simulink model "lock_srw_vA_mac"  (R2019a)
settings: Solver=VariableStepAuto  StartTime=0.0  StopTime=inf  RelTol=1e-3
undefined symbols (not defined in the file): f
libraries: dspnetwork x9, instrumentlib x9, simulink x2
(part 1 of 2)
settings Model: EnablePacing=on  PacingRate=200  Creator=SueAnne  LastModifiedBy=sheltonwright
settings DataIOCC: ReturnWorkspaceOutputs=off
settings DebuggingCC: PregeneratedLibrarySubsystemCodeDiagnostic=none  ArithmeticOperatorsInVariantConditions=warning
settings SFSimCC: SimUseLocalCustomCode=off
settings RTWCC: RTWUseLocalCustomCode=off

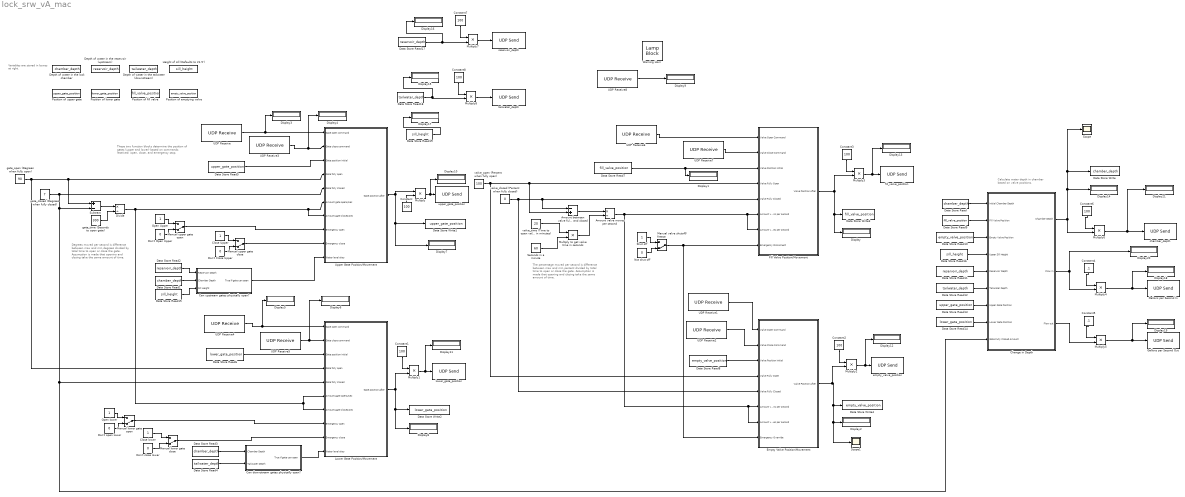
== system lock_srw_vA_mac ==
  note: These two function blocks determine the position of gates (upper and lower) based on commands received: open, close, and emergency stop.
  note: Variables are stored in boxes at right.
  note: Calculate water depth in chamber based on valve positions.
  note: Degrees moved per second is difference between max and min degrees divided by total time to open or close the gate. Assumption is made that opening and closing take the same amount of time.
  note: The percentage moved per second is difference between max and min percent divided by total time to open or close the gate. Assumption is made that opening and closing take the same amount of time.
  Amount between valve fully open and closed : Sum  Inputs=-+  OutDataTypeStr=uint8
  Amount valve moves per second : Product  Inputs=*/  OutDataTypeStr=double
  Can downstream gates physically open? : Subsystem
  Can upstream gates physically open? : Subsystem
  Change in Depth : Subsystem
  Close Upper : Constant
  Close lower : Constant
  Constant{,1..3,6..8} (7 alike) : Constant  Value=100
  Constant4 : Constant  Value=.1
  Constant5 : Constant  Value=.1
  Data Store Read : DataStoreRead  DataStoreName=chamber_depth
  Data Store Read1 : DataStoreRead  Priority=0  DataStoreName=chamber_depth
  Data Store Read10 : DataStoreRead  DataStoreName=empty_valve_position
  Data Store Read11 : DataStoreRead  DataStoreName=reservoir_depth
  Data Store Read12 : DataStoreRead  DataStoreName=tailwater_depth
  Data Store Read13 : DataStoreRead  DataStoreName=upper_gate_position
  Data Store Read14 : DataStoreRead  DataStoreName=lower_gate_position
  Data Store Read15 : DataStoreRead  Priority=0  DataStoreName=sill_height
  Data Store Read16 : DataStoreRead  Priority=0  DataStoreName=sill_height
  Data Store Read17 : DataStoreRead  Priority=0  DataStoreName=reservoir_depth
  Data Store Read18 : DataStoreRead  Priority=0  DataStoreName=tailwater_depth
  Data Store Read19 : DataStoreRead  Priority=0  DataStoreName=sill_height
  Data Store Read2 : DataStoreRead  Priority=0  DataStoreName=reservoir_depth
  Data Store Read3 : DataStoreRead  DataStoreName=chamber_depth
  Data Store Read4 : DataStoreRead  DataStoreName=tailwater_depth
  Data Store Read5 : DataStoreRead  Priority=0  DataStoreName=upper_gate_position
  Data Store Read6 : DataStoreRead  Priority=0  DataStoreName=lower_gate_position
  Data Store Read7 : DataStoreRead  Priority=0  DataStoreName=fill_valve_position
  Data Store Read8 : DataStoreRead  Priority=0  DataStoreName=empty_valve_position
  Data Store Read9 : DataStoreRead  DataStoreName=fill_valve_position
  Data Store Write : DataStoreWrite  DataStoreName=chamber_depth
  Data Store Write1 : DataStoreWrite  Priority=9  DataStoreName=upper_gate_position
  Data Store Write2 : DataStoreWrite  Priority=9  DataStoreName=lower_gate_position
  Data Store Write3 : DataStoreWrite  Priority=9  DataStoreName=fill_valve_position
  Data Store Write4 : DataStoreWrite  Priority=9  DataStoreName=empty_valve_position
  Depth of water in the lock chamber : DataStoreMemory  DataStoreName=chamber_depth  ReadBeforeWriteMsg=warning  WriteAfterWriteMsg=warning  WriteAfterReadMsg=warning  InitialValue=49.5  ShowAdditionalParam=off
  Depth of water in the reservoir (upstream) : DataStoreMemory  DataStoreName=reservoir_depth  ReadBeforeWriteMsg=warning  WriteAfterWriteMsg=warning  WriteAfterReadMsg=warning  InitialValue=28  ShowAdditionalParam=off
  Depth of water in the tailwater (downstream) : DataStoreMemory  DataStoreName=tailwater_depth  ReadBeforeWriteMsg=warning  WriteAfterWriteMsg=warning  WriteAfterReadMsg=warning  InitialValue=27  ShowAdditionalParam=off
  Display{,1..21} (22 alike) : Display
  Divide : Product  Inputs=*/  OutDataTypeStr=double
  Don't Close Upper : Constant  Value=0
  Don't Open Upper : Constant  Value=0
  Don't close lower : Constant  Value=0
  Don't open lower : Constant  Value=0
  Empty Valve Position/Movement : Subsystem
  Fill Valve Position/Movement : Subsystem
  Gallons per Second In : dspnetwork/UDP Send  remoteURL='192.168.56.2'  remotePort=23000  localURL='0.0.0.0'  localPortSource=Automatically determine  localPort=-1  sampletime=-1  blockPlatform=[]  separateLengthPort=0
      settings: SourceProductName=DSP System Toolbox  SourceProductBaseCode=DS
  Gallons per Second Out : dspnetwork/UDP Send  remoteURL='192.168.56.2'  remotePort=23001  localURL='0.0.0.0'  localPortSource=Automatically determine  localPort=-1  sampletime=-1  blockPlatform=[]  separateLengthPort=0
      settings: SourceProductName=DSP System Toolbox  SourceProductBaseCode=DS
  Height of sill (Defaults to 21.5') : DataStoreMemory  DataStoreName=sill_height  ReadBeforeWriteMsg=warning  WriteAfterWriteMsg=warning  WriteAfterReadMsg=warning  InitialValue=21.5  ShowAdditionalParam=off
  Lower Gate Position/Movement : Subsystem
  Manual lower gate close : ManualSwitch  CurrentSetting=0
  Manual lower gate open : ManualSwitch  CurrentSetting=0
  Manual upper gate close : ManualSwitch  CurrentSetting=0
  Manual upper gate open : ManualSwitch  CurrentSetting=0
  Manual valve shutoff/ freeze : ManualSwitch  CurrentSetting=0
  Multiply{,1..8} (9 alike) : Product
  Multiply to get valve time in seconds : Product  OutDataTypeStr=uint16
  Not shut off : Constant  Value=0  OutDataTypeStr=boolean
  Open Upper : Constant
  Open lower : Constant
  Position of emptying valve : DataStoreMemory  DataStoreName=empty_valve_position  ReadBeforeWriteMsg=warning  WriteAfterWriteMsg=warning  WriteAfterReadMsg=warning  ShowAdditionalParam=off
  Position of fill valve : DataStoreMemory  DataStoreName=fill_valve_position  ReadBeforeWriteMsg=warning  WriteAfterWriteMsg=warning  WriteAfterReadMsg=warning  ShowAdditionalParam=off  OutMin=0  OutMax=100  OutDataTypeStr=double
  Position of lower gate : DataStoreMemory  DataStoreName=lower_gate_position  ReadBeforeWriteMsg=warning  WriteAfterWriteMsg=warning  WriteAfterReadMsg=warning  InitialValue=7  ShowAdditionalParam=off
  Position of upper gate : DataStoreMemory  DataStoreName=upper_gate_position  ReadBeforeWriteMsg=warning  WriteAfterWriteMsg=warning  WriteAfterReadMsg=warning  InitialValue=7  ShowAdditionalParam=off
  Scope : Scope
  Scope1 : Scope
  Seconds in a minute : Constant  Value=60  OutDataTypeStr=uint8
  Shut off : Constant  OutDataTypeStr=boolean
  Subtract : Sum  Inputs=+-
  UDP Receive : instrumentlib/UDP Receive  Host=localhost  Port=9090  LocalPort=22000  EnablePortSharing=off  GetLatestData=on  DataSize=[1 1]  DataType=uint16  ASCIIFormatting=%f,  Terminator=LF  ByteOrder=LittleEndian  EnableBlockingMode=on  Timeout=10  SampleTime=1  LocalAddress=192.168.56.1
      settings: SourceProductName=Instrument Control Toolbox
  UDP Receive1 : instrumentlib/UDP Receive  Host=localhost  Port=9090  LocalPort=22006  EnablePortSharing=off  GetLatestData=on  DataSize=[1 1]  DataType=uint16  ASCIIFormatting=%f,  Terminator=LF  ByteOrder=LittleEndian  EnableBlockingMode=on  Timeout=10  SampleTime=1  LocalAddress=192.168.56.1
      settings: SourceProductName=Instrument Control Toolbox
  UDP Receive2 : instrumentlib/UDP Receive  Host=localhost  Port=9090  LocalPort=22007  EnablePortSharing=off  GetLatestData=on  DataSize=[1 1]  DataType=uint16  ASCIIFormatting=%f,  Terminator=LF  ByteOrder=LittleEndian  EnableBlockingMode=on  Timeout=10  SampleTime=1  LocalAddress=192.168.56.1
      settings: SourceProductName=Instrument Control Toolbox
  UDP Receive3 : instrumentlib/UDP Receive  Host=localhost  Port=9090  LocalPort=22001  EnablePortSharing=off  GetLatestData=on  DataSize=[1 1]  DataType=uint16  ASCIIFormatting=%f,  Terminator=LF  ByteOrder=LittleEndian  EnableBlockingMode=on  Timeout=10  SampleTime=1  LocalAddress=192.168.56.1
      settings: SourceProductName=Instrument Control Toolbox
  UDP Receive4 : instrumentlib/UDP Receive  Host=localhost  Port=9090  LocalPort=22002  EnablePortSharing=off  GetLatestData=on  DataSize=[1 1]  DataType=uint16  ASCIIFormatting=%f,  Terminator=LF  ByteOrder=LittleEndian  EnableBlockingMode=on  Timeout=10  SampleTime=1  LocalAddress=192.168.56.1
      settings: SourceProductName=Instrument Control Toolbox
  UDP Receive5 : instrumentlib/UDP Receive  Host=localhost  Port=9090  LocalPort=22003  EnablePortSharing=off  GetLatestData=on  DataSize=[1 1]  DataType=uint16  ASCIIFormatting=%f,  Terminator=LF  ByteOrder=LittleEndian  EnableBlockingMode=on  Timeout=10  SampleTime=1  LocalAddress=192.168.56.1
      settings: SourceProductName=Instrument Control Toolbox
  UDP Receive6 : instrumentlib/UDP Receive  Host=localhost  Port=9090  LocalPort=22004  EnablePortSharing=off  GetLatestData=on  DataSize=[1 1]  DataType=uint16  ASCIIFormatting=%f,  Terminator=LF  ByteOrder=LittleEndian  EnableBlockingMode=on  Timeout=10  SampleTime=1  LocalAddress=192.168.56.1
      settings: SourceProductName=Instrument Control Toolbox
  UDP Receive7 : instrumentlib/UDP Receive  Host=localhost  Port=9090  LocalPort=22005  EnablePortSharing=off  GetLatestData=on  DataSize=[1 1]  DataType=uint16  ASCIIFormatting=%f,  Terminator=LF  ByteOrder=LittleEndian  EnableBlockingMode=on  Timeout=10  SampleTime=1  LocalAddress=192.168.56.1
      settings: SourceProductName=Instrument Control Toolbox
  UDP Receive8 : instrumentlib/UDP Receive  Host=localhost  Port=9090  LocalPort=22010  EnablePortSharing=off  GetLatestData=on  DataSize=[1 1]  DataType=uint16  ASCIIFormatting=%f,  Terminator=LF  ByteOrder=LittleEndian  EnableBlockingMode=on  Timeout=10  SampleTime=1  LocalAddress=192.168.56.1
      settings: SourceProductName=Instrument Control Toolbox
  Upper Gate Position/Movement : Subsystem
  Warning Horn : LampBlock
  chamber_depth : dspnetwork/UDP Send  remoteURL='192.168.56.2'  remotePort=23006  localURL='0.0.0.0'  localPortSource=Automatically determine  localPort=-1  sampletime=-1  blockPlatform=[]  separateLengthPort=0
      settings: SourceProductName=DSP System Toolbox  SourceProductBaseCode=DS
  empty_valve_position : dspnetwork/UDP Send  remoteURL='192.168.56.2'  remotePort=23005  localURL='0.0.0.0'  localPortSource=Automatically determine  localPort=-1  sampletime=-1  blockPlatform=[]  separateLengthPort=0
      settings: SourceProductName=DSP System Toolbox  SourceProductBaseCode=DS
  fill_valve_position : dspnetwork/UDP Send  remoteURL='192.168.56.2'  remotePort=23004  localURL='0.0.0.0'  localPortSource=Automatically determine  localPort=-1  sampletime=-1  blockPlatform=[]  separateLengthPort=0
      settings: SourceProductName=DSP System Toolbox  SourceProductBaseCode=DS
  gate_closed (Degrees when fully closed) : Constant  Value=7
  gate_open (Degrees when fully open) : Constant  Value=90
  gate_time (Seconds to open gate) : Constant  Value=300
  lower_gate_position : dspnetwork/UDP Send  remoteURL='192.168.56.2'  remotePort=23003  localURL='0.0.0.0'  localPortSource=Automatically determine  localPort=-1  sampletime=-1  blockPlatform=[]  separateLengthPort=0
      settings: SourceProductName=DSP System Toolbox  SourceProductBaseCode=DS
  reservoir_depth : dspnetwork/UDP Send  remoteURL='192.168.56.2'  remotePort=23007  localURL='0.0.0.0'  localPortSource=Automatically determine  localPort=-1  sampletime=-1  blockPlatform=[]  separateLengthPort=0
      settings: SourceProductName=DSP System Toolbox  SourceProductBaseCode=DS
  tailwater_depth : dspnetwork/UDP Send  remoteURL='192.168.56.2'  remotePort=23008  localURL='0.0.0.0'  localPortSource=Automatically determine  localPort=-1  sampletime=-1  blockPlatform=[]  separateLengthPort=0
      settings: SourceProductName=DSP System Toolbox  SourceProductBaseCode=DS
  upper_gate_position : dspnetwork/UDP Send  remoteURL='192.168.56.2'  remotePort=23002  localURL='0.0.0.0'  localPortSource=Automatically determine  localPort=-1  sampletime=-1  blockPlatform=[]  separateLengthPort=0
      settings: SourceProductName=DSP System Toolbox  SourceProductBaseCode=DS
  valve_closed (Percent when fully closed) : Constant  Value=0  OutDataTypeStr=uint8
  valve_open (Percent when fully open) : Constant  Value=100  OutDataTypeStr=uint8
  "valve_time (Time to open valve, in minutes)" : Constant  Value=20  OutDataTypeStr=uint8
  wires:
  UDP Receive/1 -> Display3/1, Upper Gate Position/Movement/1(Gate open command)
  UDP Receive3/1 -> Display4/1, Upper Gate Position/Movement/2(Gate close command)
  gate_open (Degrees when fully open)/1 -> Lower Gate Position/Movement/4(Gate fully open), Subtract/1, Upper Gate Position/Movement/4(Gate fully open)
  gate_closed (Degrees when fully closed)/1 -> Change in Depth/9(Gate Fully Closed Amount), Lower Gate Position/Movement/5(Gate fully closed), Subtract/2, Upper Gate Position/Movement/5(Gate fully closed)
  Manual upper gate open/1 -> Upper Gate Position/Movement/8(Emergency open)
  Data Store Read/1 -> Change in Depth/1(Initial Chamber Depth)
  Change in Depth/1(Chamber Depth) -> Multiply6/2, Scope/1, Data Store Write/1, Display14/1
  Lower Gate Position/Movement/1(Gate position after) -> Multiply1/2, Data Store Write2/1, Display8/1
  UDP Receive4/1 -> Lower Gate Position/Movement/1(Gate open command), Display5/1
  Can upstream gates physically open?/1(True if gate can open) -> Upper Gate Position/Movement/10(Water level okay)
  Data Store Read4/1 -> Can downstream gates physically open?/2(Tailwater Depth)
  Data Store Read3/1 -> Can downstream gates physically open?/1(Chamber Depth)
  Data Store Read1/1 -> Can upstream gates physically open?/2(Chamber Depth)
  Data Store Read5/1 -> Upper Gate Position/Movement/3(Gate position initial)
  Data Store Read6/1 -> Lower Gate Position/Movement/3(Gate position initial)
  gate_time (Seconds to open gate)/1 -> Divide/2
  Subtract/1 -> Divide/1
  Divide/1 -> Lower Gate Position/Movement/7(Amount gate closes/sec), Lower Gate Position/Movement/6(Amount gate opens/sec), Upper Gate Position/Movement/7(Amount gate closes/sec), Upper Gate Position/Movement/6(Amount gate opens/sec)
  Data Store Read7/1 -> Display1/1, Fill Valve Position/Movement/3(Valve Position Initial)
  valve_open (Percent when fully open)/1 -> Amount between valve fully open and closed/2, Fill Valve Position/Movement/4(Valve Fully Open), Empty Valve Position/Movement/4(Valve Fully Open)
  valve_closed (Percent when fully closed)/1 -> Fill Valve Position/Movement/5(Valve Fully Closed), Amount between valve fully open and closed/1, Empty Valve Position/Movement/5(Valve Fully Closed)
  Manual valve shutoff/ freeze/1 -> Fill Valve Position/Movement/8(Emergency Disconnect), Empty Valve Position/Movement/8(Emergency Override)
  "valve_time (Time to open valve, in minutes)"/1 -> Multiply to get valve time in seconds/1
  Seconds in a minute/1 -> Multiply to get valve time in seconds/2
  Amount between valve fully open and closed/1 -> Amount valve moves per second/1
  Multiply to get valve time in seconds/1 -> Amount valve moves per second/2
  Amount valve moves per second/1 -> Fill Valve Position/Movement/7(Amount valve closes per second), Fill Valve Position/Movement/6(Amount valve opens per second), Empty Valve Position/Movement/7(Amount valve closes per second), Empty Valve Position/Movement/6(Amount valve opens per second)
  Data Store Read8/1 -> Empty Valve Position/Movement/3(Valve Position Initial)
  Data Store Read9/1 -> Change in Depth/2(Fill Valve Position)
  Data Store Read10/1 -> Change in Depth/3(Empty Valve Position)
  UDP Receive6/1 -> Fill Valve Position/Movement/1(Valve Open Command)
  UDP Receive7/1 -> Fill Valve Position/Movement/2(Valve Close Command)
  UDP Receive1/1 -> Empty Valve Position/Movement/1(Valve Open Command)
  UDP Receive2/1 -> Empty Valve Position/Movement/2(Valve Close Command)
  UDP Receive5/1 -> Lower Gate Position/Movement/2(Gate close command), Display6/1
  Upper Gate Position/Movement/1(Gate position after) -> Multiply/1, Display7/1, Data Store Write1/1
  Multiply/1 -> Display10/1, upper_gate_position/1
  Constant/1 -> Multiply/2
  Multiply1/1 -> Display11/1, lower_gate_position/1
  Constant1/1 -> Multiply1/1
  Constant2/1 -> Multiply2/1
  Empty Valve Position/Movement/1(Valve Position After) -> Multiply2/2, Scope1/1, Display2/1, Data Store Write4/1
  Multiply2/1 -> Display12/1, empty_valve_position/1
  Fill Valve Position/Movement/1(Valve Position After) -> Multiply3/2, Data Store Write3/1, Display/1
  Multiply3/1 -> Display13/1, fill_valve_position/1
  Constant3/1 -> Multiply3/1
  Data Store Read11/1 -> Change in Depth/5(Reservoir Depth)
  Data Store Read16/1 -> Change in Depth/4(Upper Sill Height)
  Data Store Read12/1 -> Change in Depth/6(Tailwater Depth)
  Data Store Read13/1 -> Change in Depth/7(Upper Gate Position)
  Data Store Read14/1 -> Change in Depth/8(Lower Gate Position)
  Data Store Read2/1 -> Can upstream gates physically open?/1(Reservoir Depth)
  Data Store Read15/1 -> Can upstream gates physically open?/3(Sill Height)
  Don't Open Upper/1 -> Manual upper gate open/2
  Open Upper/1 -> Manual upper gate open/1
  Don't Close Upper/1 -> Manual upper gate close/2
  Manual upper gate close/1 -> Upper Gate Position/Movement/9(Emergency close)
  Close Upper/1 -> Manual upper gate close/1
  Can downstream gates physically open?/1(True if gate can open) -> Lower Gate Position/Movement/10(Water level okay)
  Don't open lower/1 -> Manual lower gate open/2
  Manual lower gate open/1 -> Lower Gate Position/Movement/8(Emergency open)
  Manual lower gate close/1 -> Lower Gate Position/Movement/9(Emergency close)
  Open lower/1 -> Manual lower gate open/1
  Close lower/1 -> Manual lower gate close/1
  Don't close lower/1 -> Manual lower gate close/2
  Shut off/1 -> Manual valve shutoff/ freeze/1
  Not shut off/1 -> Manual valve shutoff/ freeze/2
  Change in Depth/2(Flow in) -> Display20/1, Multiply4/2
  Constant4/1 -> Multiply4/1
  Multiply4/1 -> Display18/1, Gallons per Second In/1
  Constant5/1 -> Multiply5/1
  Multiply5/1 -> Display19/1, Gallons per Second Out/1
  Change in Depth/3(Flow out) -> Multiply5/2
  Data Store Read17/1 -> Display16/1, Multiply7/2
  Data Store Read18/1 -> Display15/1, Multiply8/2
  Data Store Read19/1 -> Display17/1
  UDP Receive8/1 -> Display9/1
  Constant6/1 -> Multiply6/1
  Multiply6/1 -> Display21/1, chamber_depth/1
  Constant7/1 -> Multiply7/1
  Multiply7/1 -> reservoir_depth/1
  Constant8/1 -> Multiply8/1
  Multiply8/1 -> tailwater_depth/1

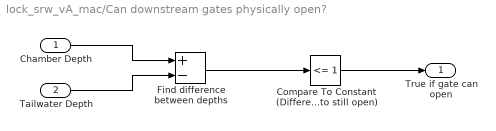
== system lock_srw_vA_mac/Can downstream gates physically open? ==
  Chamber Depth : Inport
  Tailwater Depth : Inport  Port=2
  Compare To Constant (Difference allowed between depths for gate to still open) : simulink/Logic and Bit Operations/Compare To Constant  relop=<=  const=1  OutDataTypeStr=boolean
  Find difference between depths : Sum  Inputs=+-
  True if gate can open : Outport
  wires:
  Chamber Depth/1 -> Find difference between depths/1
  Tailwater Depth/1 -> Find difference between depths/2
  Compare To Constant (Difference allowed between depths for gate to still open)/1 -> True if gate can open/1
  Find difference between depths/1 -> Compare To Constant (Difference allowed between depths for gate to still open)/1

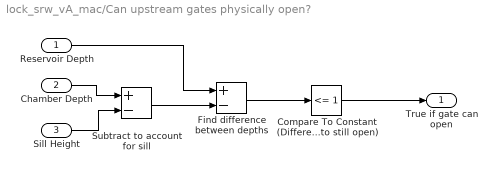
== system lock_srw_vA_mac/Can upstream gates physically open? ==
  Reservoir Depth : Inport
  Chamber Depth : Inport  Port=2
  Sill Height : Inport  Port=3
  Compare To Constant (Difference allowed between depths for gate to still open) : simulink/Logic and Bit Operations/Compare To Constant  relop=<=  const=1  OutDataTypeStr=boolean
  Find difference between depths : Sum  Inputs=+-
  Subtract to account for sill : Sum  Inputs=+-
  True if gate can open : Outport
  wires:
  Compare To Constant (Difference allowed between depths for gate to still open)/1 -> True if gate can open/1
  Find difference between depths/1 -> Compare To Constant (Difference allowed between depths for gate to still open)/1
  Subtract to account for sill/1 -> Find difference between depths/2
  Chamber Depth/1 -> Subtract to account for sill/1
  Sill Height/1 -> Subtract to account for sill/2
  Reservoir Depth/1 -> Find difference between depths/1

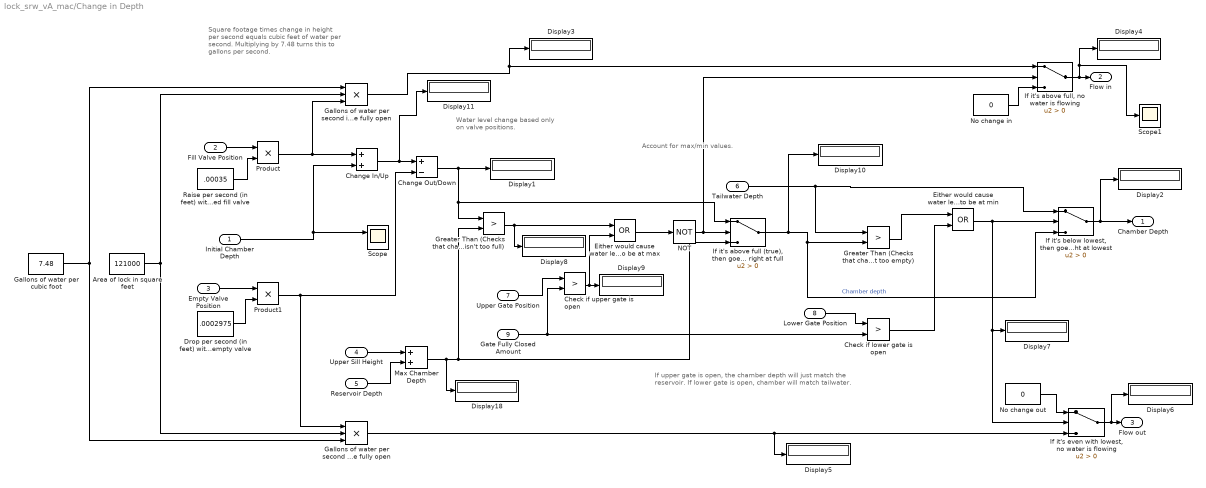
== system lock_srw_vA_mac/Change in Depth ==
  note: If upper gate is open, the chamber depth will just match the reservoir. If lower gate is open, chamber will match tailwater.
  note: Water level change based only on valve positions.
  note: Account for max/min values.
  note: Square footage times change in height per second equals cubic feet of water per second. Multiplying by 7.48 turns this to gallons per second.
  Initial Chamber Depth : Inport
  Fill Valve Position : Inport  Port=2
  Empty Valve Position : Inport  Port=3
  Upper Sill Height : Inport  Port=4
  Reservoir Depth : Inport  Port=5
  Tailwater Depth : Inport  Port=6
  Upper Gate Position : Inport  Port=7
  Lower Gate Position : Inport  Port=8
  Gate Fully Closed Amount : Inport  Port=9
  Area of lock in square feet : Constant  Value=121000  OutDataTypeStr=double
  Change Out/Down : Sum  Inputs=+-
  Change In/Up : Sum
  Check if lower gate is open : RelationalOperator  Operator=>  OutDataTypeStr=boolean  RndMeth=Simplest
  Check if upper gate is open : RelationalOperator  Operator=>  OutDataTypeStr=boolean  RndMeth=Simplest
  Display{1..11,18} (12 alike) : Display
  Drop per second (in feet) with fully opened empty valve : Constant  Value=.0002975  OutDataTypeStr=double
  Either would cause water level to be at max : Logic  Operator=OR  AllPortsSameDT=off  OutDataTypeStr=boolean
  Either would cause water level to be at min : Logic  Operator=OR  AllPortsSameDT=off  OutDataTypeStr=boolean
  Gallons of water per cubic foot : Constant  Value=7.48  OutDataTypeStr=double
  "Gallons of water per second in, when fill valve fully open" : Product  Inputs=3
  "Gallons of water per second out, when empty valve fully open" : Product  Inputs=3
  Greater Than (Checks that chamber isn't too empty) : RelationalOperator  Operator=>  OutDataTypeStr=boolean  RndMeth=Simplest
  Greater Than (Checks that chamber isn't too full) : RelationalOperator  Operator=>  OutDataTypeStr=boolean  RndMeth=Simplest
  "If it's above full (true), then goes back to being right at full" : Switch  Criteria=u2 > Threshold
  "If it's above full, no water is flowing" : Switch  Criteria=u2 > Threshold
  "If it's below lowest, then goes back to being right at lowest" : Switch  Criteria=u2 > Threshold
  "If it's even with lowest, no water is flowing" : Switch  Criteria=u2 > Threshold
  Max Chamber Depth : Sum
  NOT : Logic  Operator=NOT  IconShape=distinctive  AllPortsSameDT=off  OutDataTypeStr=boolean
  No change in : Constant  Value=0  OutDataTypeStr=double
  No change out : Constant  Value=0  OutDataTypeStr=double
  Product : Product
  Product1 : Product
  Raise per second (in feet) with fully opened fill valve : Constant  Value=.00035  OutDataTypeStr=double
  Scope : Scope  NumInputPorts=2
  Scope1 : Scope
  Chamber Depth : Outport
  Flow in : Outport  Port=2
  Flow out : Outport  Port=3
  wires:
  Fill Valve Position/1 -> Product/1
  Product/1 -> "Gallons of water per second in, when fill valve fully open"/3, Change In/Up/1
  Change In/Up/1 -> Display11/1, Change Out/Down/1
  Empty Valve Position/1 -> Product1/1
  Product1/1 -> "Gallons of water per second out, when empty valve fully open"/1, Change Out/Down/2
  Upper Sill Height/1 -> Max Chamber Depth/1
  Reservoir Depth/1 -> Max Chamber Depth/2
  Max Chamber Depth/1 -> Display18/1, Greater Than (Checks that chamber isn't too full)/2, "If it's above full (true), then goes back to being right at full"/3
  Change Out/Down/1 -> "If it's above full (true), then goes back to being right at full"/1, Greater Than (Checks that chamber isn't too full)/1, Display1/1
  "If it's above full (true), then goes back to being right at full"/1 -> Display10/1, Greater Than (Checks that chamber isn't too empty)/2, "If it's below lowest, then goes back to being right at lowest"/3  "Chamber depth"
  Greater Than (Checks that chamber isn't too full)/1 -> Either would cause water level to be at max/1, Display8/1
  Upper Gate Position/1 -> Check if upper gate is open/1
  Gate Fully Closed Amount/1 -> Check if upper gate is open/2, Check if lower gate is open/2
  Greater Than (Checks that chamber isn't too empty)/1 -> Either would cause water level to be at min/1
  Either would cause water level to be at min/1 -> Display7/1, "If it's even with lowest, no water is flowing"/2, "If it's below lowest, then goes back to being right at lowest"/2
  Lower Gate Position/1 -> Check if lower gate is open/1
  "If it's below lowest, then goes back to being right at lowest"/1 -> Display2/1, Chamber Depth/1
  Check if upper gate is open/1 -> Either would cause water level to be at max/2, Display9/1
  Gallons of water per cubic foot/1 -> "Gallons of water per second in, when fill valve fully open"/1, "Gallons of water per second out, when empty valve fully open"/3
  Initial Chamber Depth/1 -> Scope/1, Change In/Up/2
  Drop per second (in feet) with fully opened empty valve/1 -> Product1/2
  Raise per second (in feet) with fully opened fill valve/1 -> Product/2
  Area of lock in square feet/1 -> "Gallons of water per second out, when empty valve fully open"/2, "Gallons of water per second in, when fill valve fully open"/2
  "Gallons of water per second in, when fill valve fully open"/1 -> "If it's above full, no water is flowing"/1, Display3/1
  "If it's above full, no water is flowing"/1 -> Display4/1, Scope1/1, Flow in/1
  No change in/1 -> "If it's above full, no water is flowing"/3
  "If it's even with lowest, no water is flowing"/1 -> Flow out/1, Display6/1
  "Gallons of water per second out, when empty valve fully open"/1 -> Display5/1, "If it's even with lowest, no water is flowing"/3
  Tailwater Depth/1 -> Greater Than (Checks that chamber isn't too empty)/1, "If it's below lowest, then goes back to being right at lowest"/1
  No change out/1 -> "If it's even with lowest, no water is flowing"/1
  Either would cause water level to be at max/1 -> NOT/1
  NOT/1 -> "If it's above full, no water is flowing"/2, "If it's above full (true), then goes back to being right at full"/2
  Check if lower gate is open/1 -> Either would cause water level to be at min/2

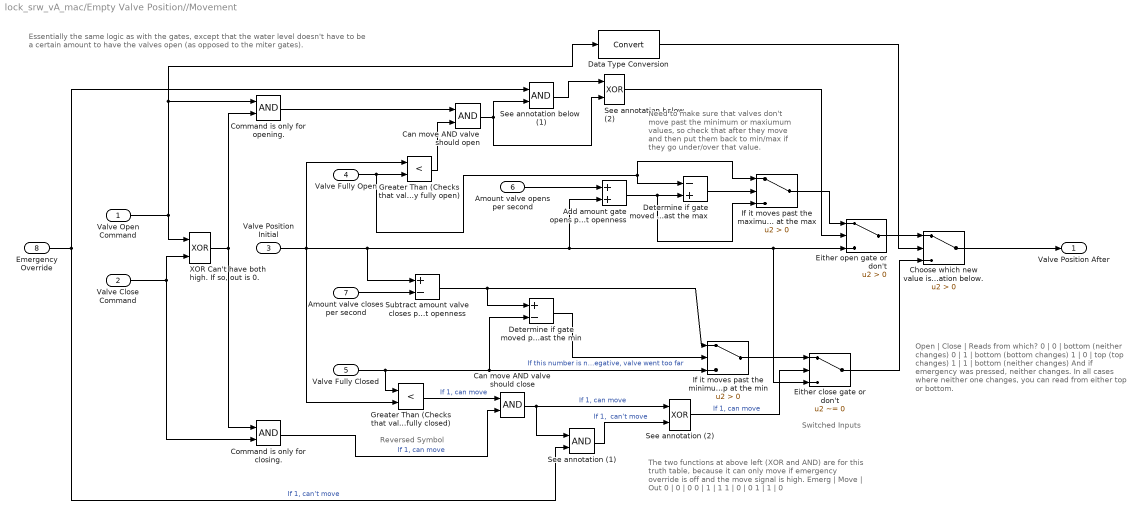
== system lock_srw_vA_mac/Empty Valve Position//Movement ==
  note: Switched Inputs
  note: Reversed Symbol
  note: Essentially the same logic as with the gates, except that the water level doesn't have to be a certain amount to have the valves open (as opposed to the miter gates).
  note: Open	|	Close	|	Reads from which?
      | 0		|	0		|	bottom (neither changes)
      | 0		|	1		|	bottom (bottom changes)
      | 1		|	0		|	top (top changes)
      | 1		|	1		|	bottom (neither changes)
      |
      | And if emergency was pressed, neither changes.  In all cases where neither one changes, you can read from either top or bottom.
  note: The two functions at above left (XOR and AND) are for this truth table, because it can only move if emergency override is off and the move signal is high.
      |
      | Emerg	|	Move	| Out
      | 0		|	0		|	0
      | 0		|	1		|	1
      | 1		|	0		|	0
      | 1		|	1		|	0
  note: Need to make sure that valves don't move past the minimum or maxiumum values, so check that after they move and then put them back to min/max if they go under/over that value.
  Valve Open Command : Inport
  Valve Close Command : Inport  Port=2
  Valve Position Initial : Inport  Port=3
  Valve Fully Open : Inport  Port=4
  Valve Fully Closed : Inport  Port=5
  Amount valve opens per second : Inport  Port=6
  Amount valve closes per second : Inport  Port=7
  Emergency Override : Inport  Port=8
  Add amount gate opens per second to current openness : Sum
  Can move AND valve should close : Logic  AllPortsSameDT=off  OutDataTypeStr=boolean
  Can move AND valve should open : Logic  AllPortsSameDT=off  OutDataTypeStr=boolean
  "Choose which new value is correct, based upon the open command. See annotation below." : Switch  Criteria=u2 > Threshold
  Command is only for closing. : Logic  AllPortsSameDT=off  OutDataTypeStr=boolean
  Command is only for opening. : Logic  AllPortsSameDT=off  OutDataTypeStr=boolean
  Data Type Conversion : DataTypeConversion
  Determine if gate moved past the max : Sum  Inputs=-+
  Determine if gate moved past the min : Sum  Inputs=+-
  Either close gate or don't : Switch  Criteria=u2 ~= 0  RndMeth=Simplest
  Either open gate or don't : Switch  Criteria=u2 > Threshold
  Greater Than (Checks that valve isn't already fully closed) : RelationalOperator  Operator=<  OutDataTypeStr=boolean  RndMeth=Simplest
  Greater Than (Checks that valve isn't already fully open) : RelationalOperator  Operator=<  OutDataTypeStr=boolean  RndMeth=Simplest
  "If it moves past the maximum, it will stop at the max" : Switch  Criteria=u2 > Threshold
  "If it moves past the minimum, it will stop at the min" : Switch  Criteria=u2 > Threshold
  See annotation below  (1) : Logic  AllPortsSameDT=off  OutDataTypeStr=boolean
  See annotation below (2) : Logic  Operator=XOR  IconShape=distinctive  AllPortsSameDT=off  OutDataTypeStr=boolean
  See annotation (1) : Logic  AllPortsSameDT=off  OutDataTypeStr=boolean
  See annotation (2) : Logic  Operator=XOR  IconShape=distinctive  AllPortsSameDT=off  OutDataTypeStr=boolean
  Subtract amount valve closes per second from current openness : Sum  Inputs=+-
  "XOR Can't have both high. If so, out is 0." : Logic  Operator=XOR  IconShape=distinctive  AllPortsSameDT=off  OutDataTypeStr=boolean
  Valve Position After : Outport
  wires:
  Command is only for opening./1 -> Can move AND valve should open/1
  Greater Than (Checks that valve isn't already fully open)/1 -> Can move AND valve should open/2
  Either open gate or don't/1 -> "Choose which new value is correct, based upon the open command. See annotation below."/1
  See annotation (1)/1 -> See annotation (2)/2  "If 1,  can't move"
  Valve Open Command/1 -> Data Type Conversion/1, Command is only for opening./1, "XOR Can't have both high. If so, out is 0."/1
  Valve Fully Open/1 -> Determine if gate moved past the max/1, "If it moves past the maximum, it will stop at the max"/1, Greater Than (Checks that valve isn't already fully open)/2
  "If it moves past the maximum, it will stop at the max"/1 -> Either open gate or don't/1
  Subtract amount valve closes per second from current openness/1 -> "If it moves past the minimum, it will stop at the min"/1, Determine if gate moved past the min/1
  Can move AND valve should open/1 -> See annotation below (2)/2, See annotation below  (1)/2
  Amount valve closes per second/1 -> Subtract amount valve closes per second from current openness/2
  See annotation below  (1)/1 -> See annotation below (2)/1
  Valve Position Initial/1 -> Greater Than (Checks that valve isn't already fully open)/1, Either close gate or don't/3, Either open gate or don't/3, Add amount gate opens per second to current openness/2, Subtract amount valve closes per second from current openness/1, Greater Than (Checks that valve isn't already fully closed)/2
  Either close gate or don't/1 -> "Choose which new value is correct, based upon the open command. See annotation below."/3
  Emergency Override/1 -> See annotation below  (1)/1, See annotation (1)/2  "If 1, can't move"
  See annotation below (2)/1 -> Either open gate or don't/2
  Valve Close Command/1 -> Command is only for closing./2, "XOR Can't have both high. If so, out is 0."/2
  Command is only for closing./1 -> Can move AND valve should close/2  "If 1, can move"
  See annotation (2)/1 -> Either close gate or don't/2  "If 1, can move"
  Can move AND valve should close/1 -> See annotation (2)/1, See annotation (1)/1  "If 1, can move"
  Add amount gate opens per second to current openness/1 -> Determine if gate moved past the max/2, "If it moves past the maximum, it will stop at the max"/3
  Determine if gate moved past the min/1 -> "If it moves past the minimum, it will stop at the min"/2  "If this number is negative, valve went too far"
  Greater Than (Checks that valve isn't already fully closed)/1 -> Can move AND valve should close/1  "If 1, can move"
  Valve Fully Closed/1 -> "If it moves past the minimum, it will stop at the min"/3, Determine if gate moved past the min/2, Greater Than (Checks that valve isn't already fully closed)/1
  Determine if gate moved past the max/1 -> "If it moves past the maximum, it will stop at the max"/2
  "XOR Can't have both high. If so, out is 0."/1 -> Command is only for closing./1, Command is only for opening./2
  Amount valve opens per second/1 -> Add amount gate opens per second to current openness/1
  "Choose which new value is correct, based upon the open command. See annotation below."/1 -> Valve Position After/1
  Data Type Conversion/1 -> "Choose which new value is correct, based upon the open command. See annotation below."/2
  "If it moves past the minimum, it will stop at the min"/1 -> Either close gate or don't/1

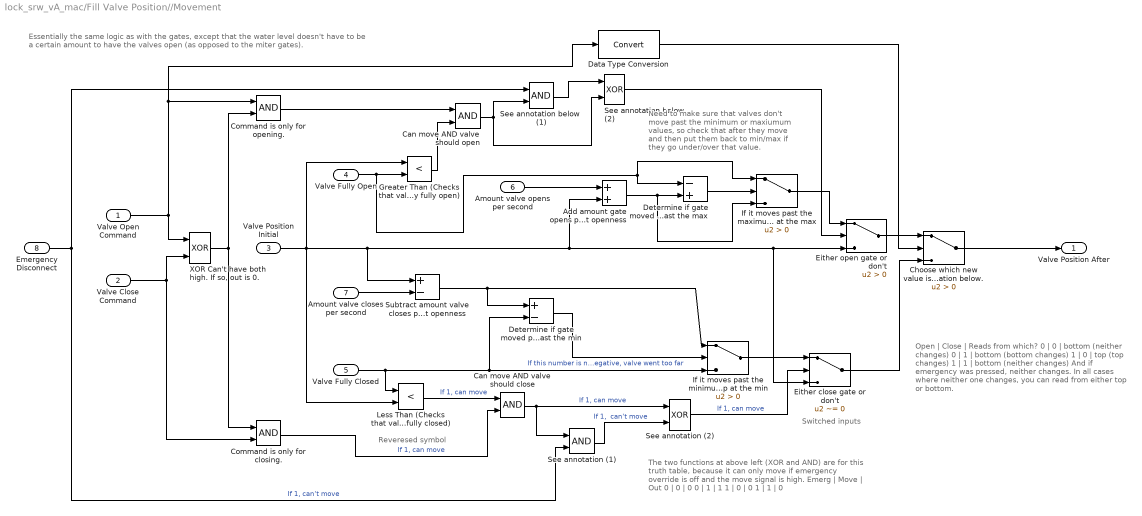
== system lock_srw_vA_mac/Fill Valve Position//Movement ==
  note: Switched inputs
  note: Reveresed symbol
  note: Essentially the same logic as with the gates, except that the water level doesn't have to be a certain amount to have the valves open (as opposed to the miter gates).
  note: Open	|	Close	|	Reads from which?
      | 0		|	0		|	bottom (neither changes)
      | 0		|	1		|	bottom (bottom changes)
      | 1		|	0		|	top (top changes)
      | 1		|	1		|	bottom (neither changes)
      |
      | And if emergency was pressed, neither changes.  In all cases where neither one changes, you can read from either top or bottom.
  note: The two functions at above left (XOR and AND) are for this truth table, because it can only move if emergency override is off and the move signal is high.
      |
      | Emerg	|	Move	| Out
      | 0		|	0		|	0
      | 0		|	1		|	1
      | 1		|	0		|	0
      | 1		|	1		|	0
  note: Need to make sure that valves don't move past the minimum or maxiumum values, so check that after they move and then put them back to min/max if they go under/over that value.
  Valve Open Command : Inport
  Valve Close Command : Inport  Port=2
  Valve Position Initial : Inport  Port=3
  Valve Fully Open : Inport  Port=4
  Valve Fully Closed : Inport  Port=5
  Amount valve opens per second : Inport  Port=6
  Amount valve closes per second : Inport  Port=7
  Emergency Disconnect : Inport  Port=8
  Add amount gate opens per second to current openness : Sum
  Can move AND valve should close : Logic  AllPortsSameDT=off  OutDataTypeStr=boolean
  Can move AND valve should open : Logic  AllPortsSameDT=off  OutDataTypeStr=boolean
  "Choose which new value is correct, based upon the open command. See annotation below." : Switch  Criteria=u2 > Threshold
  Command is only for closing. : Logic  AllPortsSameDT=off  OutDataTypeStr=boolean
  Command is only for opening. : Logic  AllPortsSameDT=off  OutDataTypeStr=boolean
  Data Type Conversion : DataTypeConversion
  Determine if gate moved past the max : Sum  Inputs=-+
  Determine if gate moved past the min : Sum  Inputs=+-
  Either close gate or don't : Switch  Criteria=u2 ~= 0  RndMeth=Simplest
  Either open gate or don't : Switch  Criteria=u2 > Threshold
  Greater Than (Checks that valve isn't already fully open) : RelationalOperator  Operator=<  OutDataTypeStr=boolean  RndMeth=Simplest
  "If it moves past the maximum, it will stop at the max" : Switch  Criteria=u2 > Threshold
  "If it moves past the minimum, it will stop at the min" : Switch  Criteria=u2 > Threshold
  Less Than (Checks that valve isn't already fully closed) : RelationalOperator  Operator=<  OutDataTypeStr=boolean  RndMeth=Simplest
  See annotation below  (1) : Logic  AllPortsSameDT=off  OutDataTypeStr=boolean
  See annotation below (2) : Logic  Operator=XOR  IconShape=distinctive  AllPortsSameDT=off  OutDataTypeStr=boolean
  See annotation (1) : Logic  AllPortsSameDT=off  OutDataTypeStr=boolean
  See annotation (2) : Logic  Operator=XOR  IconShape=distinctive  AllPortsSameDT=off  OutDataTypeStr=boolean
  Subtract amount valve closes per second from current openness : Sum  Inputs=+-
  "XOR Can't have both high. If so, out is 0." : Logic  Operator=XOR  IconShape=distinctive  AllPortsSameDT=off  OutDataTypeStr=boolean
  Valve Position After : Outport
  wires:
  Command is only for opening./1 -> Can move AND valve should open/1
  Greater Than (Checks that valve isn't already fully open)/1 -> Can move AND valve should open/2
  Either open gate or don't/1 -> "Choose which new value is correct, based upon the open command. See annotation below."/1
  See annotation (1)/1 -> See annotation (2)/2  "If 1,  can't move"
  Valve Open Command/1 -> Data Type Conversion/1, Command is only for opening./1, "XOR Can't have both high. If so, out is 0."/1
  Valve Fully Open/1 -> Determine if gate moved past the max/1, "If it moves past the maximum, it will stop at the max"/1, Greater Than (Checks that valve isn't already fully open)/2
  "If it moves past the maximum, it will stop at the max"/1 -> Either open gate or don't/1
  Subtract amount valve closes per second from current openness/1 -> "If it moves past the minimum, it will stop at the min"/1, Determine if gate moved past the min/1
  Can move AND valve should open/1 -> See annotation below (2)/2, See annotation below  (1)/2
  Amount valve closes per second/1 -> Subtract amount valve closes per second from current openness/2
  See annotation below  (1)/1 -> See annotation below (2)/1
  Valve Position Initial/1 -> Greater Than (Checks that valve isn't already fully open)/1, Either close gate or don't/3, Either open gate or don't/3, Add amount gate opens per second to current openness/2, Subtract amount valve closes per second from current openness/1, Less Than (Checks that valve isn't already fully closed)/2
  Either close gate or don't/1 -> "Choose which new value is correct, based upon the open command. See annotation below."/3
  Emergency Disconnect/1 -> See annotation below  (1)/1, See annotation (1)/2  "If 1, can't move"
  See annotation below (2)/1 -> Either open gate or don't/2
  Valve Close Command/1 -> Command is only for closing./2, "XOR Can't have both high. If so, out is 0."/2
  Command is only for closing./1 -> Can move AND valve should close/2  "If 1, can move"
  Can move AND valve should close/1 -> See annotation (2)/1, See annotation (1)/1  "If 1, can move"
  Add amount gate opens per second to current openness/1 -> Determine if gate moved past the max/2, "If it moves past the maximum, it will stop at the max"/3
  Determine if gate moved past the min/1 -> "If it moves past the minimum, it will stop at the min"/2  "If this number is negative, valve went too far"
  Less Than (Checks that valve isn't already fully closed)/1 -> Can move AND valve should close/1  "If 1, can move"
  Valve Fully Closed/1 -> "If it moves past the minimum, it will stop at the min"/3, Determine if gate moved past the min/2, Less Than (Checks that valve isn't already fully closed)/1
  Determine if gate moved past the max/1 -> "If it moves past the maximum, it will stop at the max"/2
  "XOR Can't have both high. If so, out is 0."/1 -> Command is only for closing./1, Command is only for opening./2
  Amount valve opens per second/1 -> Add amount gate opens per second to current openness/1
  "Choose which new value is correct, based upon the open command. See annotation below."/1 -> Valve Position After/1
  Data Type Conversion/1 -> "Choose which new value is correct, based upon the open command. See annotation below."/2
  See annotation (2)/1 -> Either close gate or don't/2  "If 1, can move"
  "If it moves past the minimum, it will stop at the min"/1 -> Either close gate or don't/1

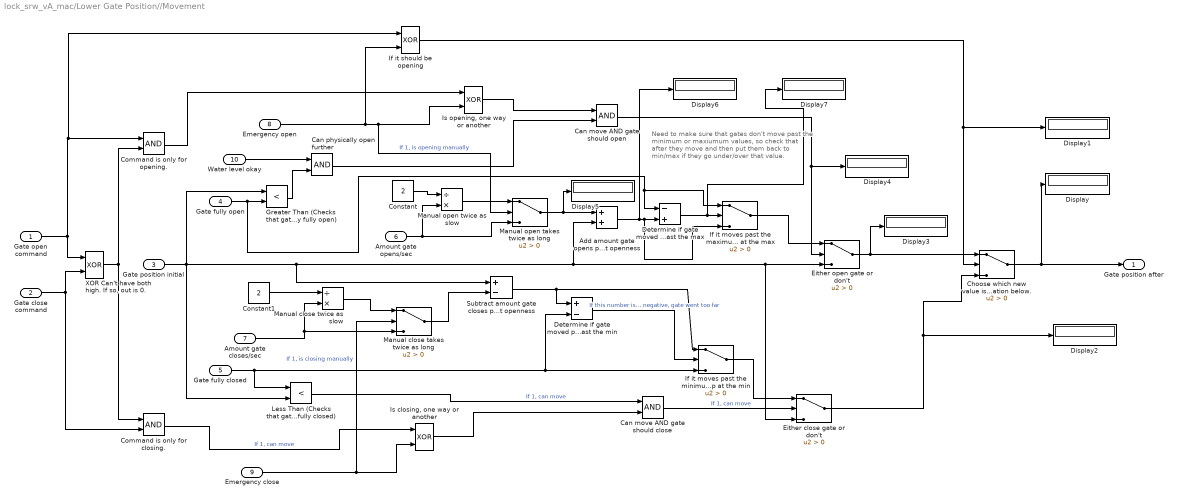
== system lock_srw_vA_mac/Lower Gate Position//Movement ==
  note: Need to make sure that gates don't move past the minimum or maxiumum values, so check that after they move and then put them back to min/max if they go under/over that value.
  Gate open command : Inport
  Gate close command : Inport  Port=2
  Gate position initial : Inport  Port=3
  Gate fully open : Inport  Port=4
  Gate fully closed : Inport  Port=5
  Amount gate opens/sec : Inport  Port=6
  Amount gate closes/sec : Inport  Port=7
  Emergency open : Inport  Port=8
  Emergency close : Inport  Port=9
  Water level okay : Inport  Port=10
  Add amount gate opens per second to current openness : Sum
  Can move AND gate should close : Logic  AllPortsSameDT=off  OutDataTypeStr=boolean
  Can move AND gate should open : Logic  AllPortsSameDT=off  OutDataTypeStr=boolean
  Can physically open further : Logic  AllPortsSameDT=off  OutDataTypeStr=boolean
  "Choose which new value is correct, based upon the open command. See annotation below." : Switch  Criteria=u2 > Threshold
  Command is only for closing. : Logic  AllPortsSameDT=off  OutDataTypeStr=boolean
  Command is only for opening. : Logic  AllPortsSameDT=off  OutDataTypeStr=boolean
  Constant : Constant  Value=2
  Constant1 : Constant  Value=2
  Determine if gate moved past the max : Sum  Inputs=-+
  Determine if gate moved past the min : Sum  Inputs=+-
  Display{,1..7} (8 alike) : Display
  Either close gate or don't : Switch  Criteria=u2 > Threshold
  Either open gate or don't : Switch  Criteria=u2 > Threshold
  Greater Than (Checks that gate isn't already fully open) : RelationalOperator  Operator=<  OutDataTypeStr=boolean  RndMeth=Simplest
  "If it moves past the maximum, it will stop at the max" : Switch  Criteria=u2 > Threshold
  "If it moves past the minimum, it will stop at the min" : Switch  Criteria=u2 > Threshold
  If it should be opening : Logic  Operator=XOR  IconShape=distinctive  AllPortsSameDT=off  OutDataTypeStr=boolean
  "Is closing, one way or another" : Logic  Operator=XOR  IconShape=distinctive  AllPortsSameDT=off  OutDataTypeStr=boolean
  "Is opening, one way or another" : Logic  Operator=XOR  IconShape=distinctive  AllPortsSameDT=off  OutDataTypeStr=boolean
  Less Than (Checks that gate isn't already fully closed) : RelationalOperator  Operator=<  OutDataTypeStr=boolean  RndMeth=Simplest
  Manual close takes twice as long : Switch  Criteria=u2 > Threshold
  Manual close twice as slow : Product  Inputs=/*
  Manual open takes twice as long : Switch  Criteria=u2 > Threshold
  Manual open twice as slow : Product  Inputs=/*
  Subtract amount gate closes per second from current openness : Sum  Inputs=+-
  "XOR Can't have both high. If so, out is 0." : Logic  Operator=XOR  IconShape=distinctive  AllPortsSameDT=off  OutDataTypeStr=boolean
  Gate position after : Outport
  wires:
  Gate open command/1 -> If it should be opening/1, Command is only for opening./1, "XOR Can't have both high. If so, out is 0."/1
  Gate close command/1 -> Command is only for closing./2, "XOR Can't have both high. If so, out is 0."/2
  "XOR Can't have both high. If so, out is 0."/1 -> Command is only for closing./1, Command is only for opening./2
  Gate position initial/1 -> Greater Than (Checks that gate isn't already fully open)/1, Either open gate or don't/3, Either close gate or don't/3, Add amount gate opens per second to current openness/2, Subtract amount gate closes per second from current openness/1, Less Than (Checks that gate isn't already fully closed)/2
  "Choose which new value is correct, based upon the open command. See annotation below."/1 -> Display/1, Gate position after/1
  Can move AND gate should close/1 -> Either close gate or don't/2  "If 1, can move"
  Either open gate or don't/1 -> Display3/1, "Choose which new value is correct, based upon the open command. See annotation below."/1
  Either close gate or don't/1 -> "Choose which new value is correct, based upon the open command. See annotation below."/3, Display2/1
  Greater Than (Checks that gate isn't already fully open)/1 -> Can physically open further/2
  Can physically open further/1 -> Can move AND gate should open/2
  Less Than (Checks that gate isn't already fully closed)/1 -> Can move AND gate should close/1  "If 1, can move"
  Water level okay/1 -> Can physically open further/1
  Can move AND gate should open/1 -> Display4/1, Either open gate or don't/2
  Gate fully closed/1 -> "If it moves past the minimum, it will stop at the min"/3, Determine if gate moved past the min/2, Less Than (Checks that gate isn't already fully closed)/1
  "If it moves past the minimum, it will stop at the min"/1 -> Either close gate or don't/1
  Subtract amount gate closes per second from current openness/1 -> Determine if gate moved past the min/1, "If it moves past the minimum, it will stop at the min"/1
  Determine if gate moved past the min/1 -> "If it moves past the minimum, it will stop at the min"/2  "If this number is negative, gate went too far"
  Gate fully open/1 -> "If it moves past the maximum, it will stop at the max"/1, Determine if gate moved past the max/1, Greater Than (Checks that gate isn't already fully open)/2
  Determine if gate moved past the max/1 -> Display7/1, "If it moves past the maximum, it will stop at the max"/2
  "If it moves past the maximum, it will stop at the max"/1 -> Either open gate or don't/1
  Add amount gate opens per second to current openness/1 -> Display6/1, Determine if gate moved past the max/2, "If it moves past the maximum, it will stop at the max"/3
  "Is closing, one way or another"/1 -> Can move AND gate should close/2
  Emergency close/1 -> Manual close takes twice as long/2, "Is closing, one way or another"/2  "If 1, is closing manually"
  Command is only for closing./1 -> "Is closing, one way or another"/1  "If 1, can move"
  "Is opening, one way or another"/1 -> Can move AND gate should open/1
  Emergency open/1 -> If it should be opening/2, "Is opening, one way or another"/2, Manual open takes twice as long/2  "If 1, is opening manually"
  Command is only for opening./1 -> "Is opening, one way or another"/1
  Amount gate opens/sec/1 -> Manual open takes twice as long/3, Manual open twice as slow/2
  Manual open twice as slow/1 -> Manual open takes twice as long/1
  Manual open takes twice as long/1 -> Display5/1, Add amount gate opens per second to current openness/1
  Constant/1 -> Manual open twice as slow/1
  Manual close twice as slow/1 -> Manual close takes twice as long/1
  Amount gate closes/sec/1 -> Manual close twice as slow/2, Manual close takes twice as long/3
  Constant1/1 -> Manual close twice as slow/1
  Manual close takes twice as long/1 -> Subtract amount gate closes per second from current openness/2
  If it should be opening/1 -> Display1/1, "Choose which new value is correct, based upon the open command. See annotation below."/2
